simulink model "Model_Refrigeration_ON"  (R2022a)
settings: Solver=VariableStepAuto  StartTime=0.0  StopTime=properties_8(15,2)  FixedStep=properties_8(14,2)  MaxStep=properties_8(14,2)  RelTol=1e-3  AbsTol=1e-3
InitFcn:
  | tube_D = 0.02; % [m] Refrigerant tube diameter
  | duct_W = 0.4; % [m] Air duct width
  | house_L = 4.5; % [m] House length
  | house_W = 3; % [m] House width
  | house_H = 2; % [m] House height
  | roof_pitch = 0; % [deg] Roof pitch
undefined symbols (not defined in the file or in its folder): alpha_h_ratio_NE, alpha_h_ratio_NW, alpha_h_ratio_SE, alpha_h_ratio_SW, area_furniture, area_roof, area_wall_exterior_NE, area_wall_exterior_NW, area_wall_exterior_SE, area_wall_exterior_SW, area_window, cp_furniture, cp_roof, cp_wall_exterior_NE, cp_wall_exterior_NW, cp_wall_exterior_SE, cp_wall_exterior_SW, cp_window, hc_furniture_interior, hc_roof_exterior, hc_roof_interior, hc_wall_exterior_NE, hc_wall_exterior_NW, hc_wall_exterior_SE, hc_wall_exterior_SW, hc_wall_interior_NE, hc_wall_interior_NW, hc_wall_interior_SE, hc_wall_interior_SW, hc_window_exterior, hc_window_interior, k_roof, k_wall_NE, k_wall_NW, k_wall_SE, k_wall_SW, k_window, l_roof, mass_furniture, pitch_roof, properties_8, properties_9, Q_infiltration_latent, Q_infiltration_sensible, Q_latent_occupant_skin, Q_lights, Q_motor, Q_occupant, rho_roof, rho_wall_NE, rho_wall_NW, rho_wall_SE, rho_wall_SW, rho_window, SC, sigbuilder_block, T_env, T_house_init, T_init_furniture, T_set ... (+12)
libraries: fl_lib x102, nesl_utility x30, SimscapeFluids_lib x9, simulink_extras x3
(part 1 of 4)
CloseFcn:
  | try,close(h1_sscfluids_refrigeration),end
  | clear h1_sscfluids_refrigeration
  | try,close(h2_sscfluids_refrigeration),end
  | clear h2_sscfluids_refrigeration
  | try,close(h3_sscfluids_refrigeration),end
  | clear h3_sscfluids_refrigeration
  | Results
  | clear tout simlog_sscfluids_refrigeration
  | clear T_env RH_env T_house_init RH_house_init T_set
  | clear tube_D duct_W house_L house_W house_H roof_pitch
Description:
  | Refrigeration Cycle (Air Conditioning)
settings Model: Creator=The MathWorks, Inc.  LastModifiedBy=Aqib Habib
settings SolverCC: AutoScaleAbsTol=off  AlgebraicLoopSolver=TrustRegion  MaxZcPerStep=1
settings DataIOCC: ReturnWorkspaceOutputs=off
settings DebuggingCC: UnconnectedInputMsg=warning  UnconnectedOutputMsg=warning  UnconnectedLineMsg=warning  SymbolicDimsDataTypeCodeGenerationDiagnostic=none  SFMachineParentedDataDiag=warning
settings SFSimCC: CustomCodeUndefinedFunction=UseInterfaceOnly
settings RTWCC: DLArmComputeVersion=19.05
settings SimscapeCC: SimscapeLogType=all  SimscapeLogSimulationStatistics=on  SimscapeLogName=simlog_sscfluids_refrigeration  SimscapeLogDataHistory=10000

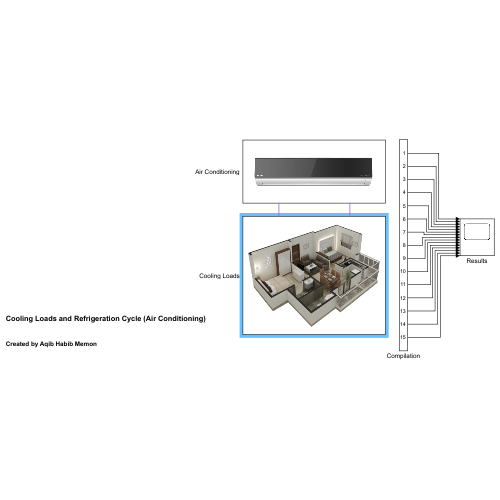
[thumbnail: Simulink's stored preview of the top-level diagram]
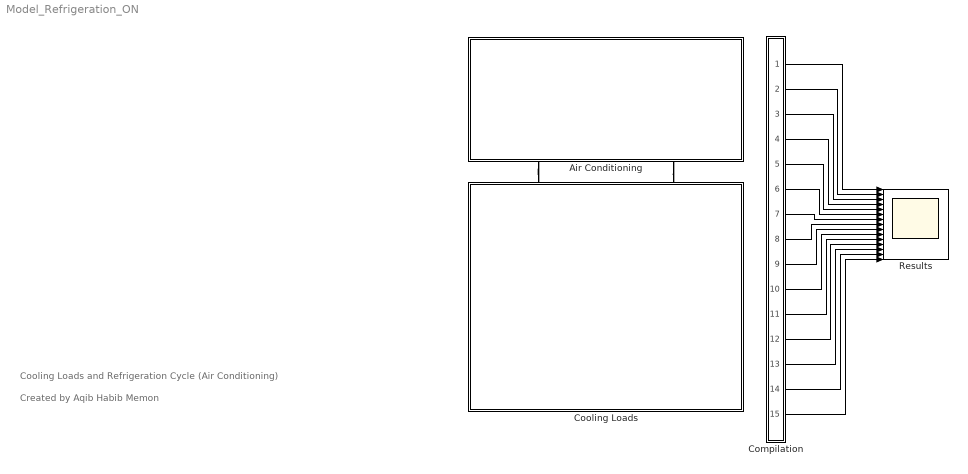
== system Model_Refrigeration_ON ==
  note: Cooling Loads and Refrigeration Cycle (Air Conditioning)
  note: Created by Aqib Habib Memon
  Air Conditioning : Subsystem
      mask Display: image('econo.png'); % Use "Edit Image" on toolstrip to change.
  Compilation : Subsystem
  Cooling Loads : Subsystem
      mask Display: image('Picture1.png'); % Use "Edit Image" on toolstrip to change.
  Results : Scope  NumInputPorts=15
  wires:
  Compilation/10(Out5) -> Results/10
  Compilation/9(Out4) -> Results/9
  Compilation/1(Out1) -> Results/1
  Compilation/2(Out13) -> Results/2
  Compilation/8(Out3) -> Results/8
  Compilation/7(Out7) -> Results/7
  Compilation/12(Out9) -> Results/12
  Compilation/5(Out2) -> Results/5
  Compilation/11(Out8) -> Results/11
  Compilation/6(Out6) -> Results/6
  Compilation/13(Out10) -> Results/13
  Compilation/3(Out12) -> Results/3
  Compilation/4(Out11) -> Results/4
  Compilation/14(Out14) -> Results/14
  Compilation/15(Out15) -> Results/15
  connections:
  Air Conditioning/RConn2 -- Cooling Loads/LConn2
  Air Conditioning/RConn1 -- Cooling Loads/LConn1

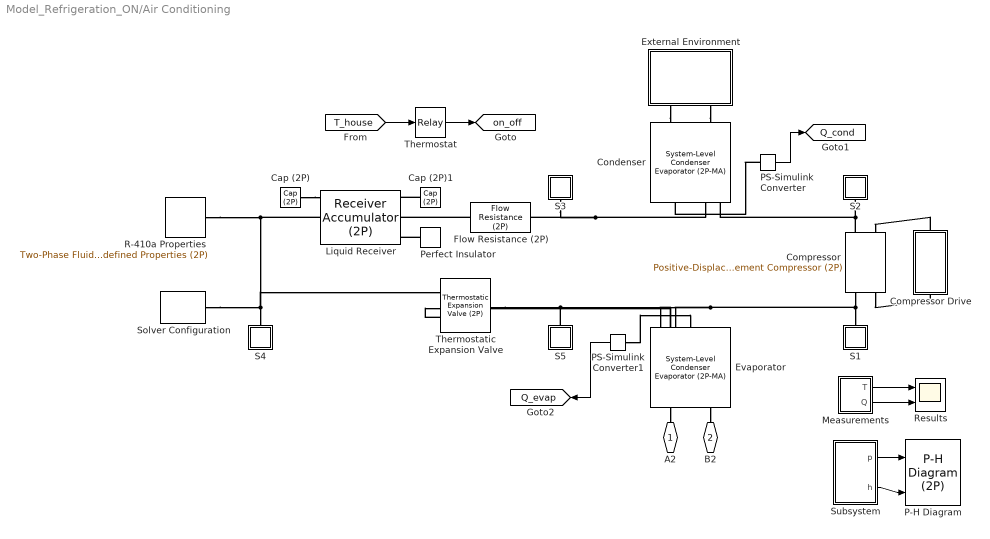
== system Model_Refrigeration_ON/Air Conditioning ==
  Cap (2P) : fl_lib/Two-Phase Fluid/Elements/Cap (2P)  p_specify=off  p_priority=None  p=0.101325 MPa  p_nominal_specify=off  p_nominal_unit=MPa  p_nominal_value=1  u_specify=off  u_priority=None  u=1500 kJ/kg  u_nominal_specify=off  u_nominal_unit=kJ/kg  u_nominal_value=1
      settings: SourceProductBaseCode=PW,SS,VE  InternalSimscapePortConfiguration="{\"Bottom\":[],\"Left\":[{\"id\":\"A\",\"label\":\"\",\"type\":\"foundation.two_phase_fluid.two_phase_fluid\"}],\"Right\":[],\"Top\":[]}"
  Cap (2P)1 : fl_lib/Two-Phase Fluid/Elements/Cap (2P)  p_specify=off  p_priority=None  p=0.101325 MPa  p_nominal_specify=off  p_nominal_unit=MPa  p_nominal_value=1  u_specify=off  u_priority=None  u=1500 kJ/kg  u_nominal_specify=off  u_nominal_unit=kJ/kg  u_nominal_value=1
      settings: SourceProductBaseCode=PW,SS,VE  InternalSimscapePortConfiguration="{\"Bottom\":[],\"Left\":[{\"id\":\"A\",\"label\":\"\",\"type\":\"foundation.two_phase_fluid.two_phase_fluid\"}],\"Right\":[],\"Top\":[]}"
  Compressor : SimscapeFluids_lib/Two-Phase Fluid/Fluid Machines/Positive-Displacement Compressor (2P)  dispSpec=fluids.two_phase_fluid.fluid_machines.enum.DisplacementSpecification.FlowSpeed  v_disp=130 cm^3/rev  mdot_nom=properties_9(1,12) kg/s  omega_nom=properties_9(2,12) rpm  nominalSpec=fluids.two_phase_fluid.fluid_machines.enum.NominalConditionsSpecification.NominalTemps  pr_nom=5  p_in_nom=0.101325 MPa  T_in_nom=373.15 K  T_evap_nom=properties_9(3,12) degC  T_cond_nom=properties_9(4,12) degC  delta_T_nom=properties_9(6,12) deltaK  efficiencySpec=fluids.two_phase_fluid.fluid_machines.enum.VolumetricEfficiencyParameterization.Analytical  eta_nom=properties_9(9,12)  omega_TLU=[800, 1500, 2800, 3300, 4000] rpm  pr_TLU=[2, 4, 6, 8]  eta_TLU=[.95, .9, .85, .8, .75; .925, .875, .825, .775, .725; .875, .825, .775, .725, .675; .75, .7, .65, .6, .55]  n=properties_9(11,12)  mechanical_efficiency=properties_9(10,12)  area_A=pi*properties_9(7,12)/4 m^2  area_B=pi*properties_9(8,12)/4 m^2  VaporCheck=simscape.enum.assert.action.none
      settings: SourceProductBaseCode=SH  InternalSimscapePortConfiguration="{\"Bottom\":[],\"Left\":[{\"id\":\"A\",\"label\":\"A\",\"type\":\"foundation.two_phase_fluid.two_phase_fluid\"},{\"id\":\"C\",\"label\":\"C\",\"type\":\"foundation.mechanical.rotational.rotational\"}],\"Right\":[{\"id\":\"B\",\"label\":\"B\",\"type\":\"foundation.two_phase_fluid.two_phase_fluid\"},{\"id\":\"R\",\"label\":\"R\",\"type\":\"foundation.mechanical.rotational.rotational\"}],\"Top\":[]}"
  Compressor Drive : Subsystem
      settings: PortSchema="{\"entries\":[{\"content\":{\"sides\":[{\"content\":{\"connectorIds\":[]},\"type\":\"ConnectorPlacement.EquallySpacedRectSide\",\"uuid\":\"e1f7673a-ae09-4e38-a748-d03f3a89f634\"},{\"content\":{\"connectorIds\":[],\"side\":\"RIGHT\"},\"type\":\"ConnectorPlacement.EquallySpacedRectSide\",\"uuid\":\"e2c59df4-5a81-4f6b-ab06-631ef800c0b1\"},{\"content\":{\"connectorIds\":[\"LConn1\"],\"side\":\"TOP\"},\"type\":\"ConnectorPlacement.EquallySpacedRectSide\",\"uuid\":\"19dd88a8-04e0-4296-a227-9de66059cdf8\"},{\"content\":{\"connectorIds\":[\"RConn1\"],\"side\":\"BOTTOM\"},\"type\":\"ConnectorPlacement.EquallySpacedRectSide\",\"uuid\":\"d46824c3-70de-4a16-8a6e-f7ccc848533a\"}]},\"type\":\"ConnectorPlacement.EquallySpacedConnector\",\"uuid\":\"cfca4f7e-9c0e-462b-910e-b09b0fceba6e\"}],\"packageUris\":[\"http://schema.mathworks.com/mf0/Connector/R2020b\"],\"version\":\"1.0\"}"
  Condenser : SimscapeFluids_lib/Fluid Network Interfaces/Heat Exchangers/System-Level Condenser Evaporator (2P-MA)  flow_arrangement=fluids.interfaces.heat_exchangers.enum.SystemLevelFlowArrangement2PMA.Cross  wall_thermal_mass=simscape.enum.onoff.off  mass_wall=1 kg  cp_wall=490 J/(K*kg)  area_A1=pi*properties_9(1,4)^2/4 m^2  area_B1=pi*properties_9(2,4)/4 m^2  area_A2=pi*properties_9(3,4)/4 m^2  area_B2=pi*properties_9(4,4)/4 m^2  operating_condition_2P=fluids.interfaces.heat_exchangers.enum.SystemLevelOperatingCondition2PMA.Condenser  mdot_nominal_2P=properties_9(11,4) kg/s  delta_p_nominal_2P=0.01 MPa  pressure_spec_cond_2P=fluids.interfaces.heat_exchangers.enum.SystemLevelPressureSpecCondenser2P.CondensingTemperature  pressure_spec_evap_2P=fluids.interfaces.heat_exchangers.enum.SystemLevelPressureSpecEvaporator2P.InletPressure  p_in_nominal_2P=1 MPa  T_cond_nominal_2P=properties_9(4,12) degC  T_evap_nominal_2P=243.15 K  inlet_spec_2P=fluids.interfaces.heat_exchangers.enum.SystemLevelInletSpec2P.Temperature  T_in_nominal_2P=properties_9(10,4) degC  h_in_nominal_2P=440 kJ/kg  x_in_nominal_2P=1  capacity_spec_2P=fluids.interfaces.heat_exchangers.enum.SystemLevelCapacitySpec.OutletCondition  Q_nominal=0.1 kW  outlet_spec_cond_2P=fluids.interfaces.heat_exchangers.enum.SystemLevelOutletSpecCondenser2P.Subcooling  outlet_spec_evap_2P=fluids.interfaces.heat_exchangers.enum.SystemLevelOutletSpecEvaporator2P.Enthalpy  delta_T_sub_nominal_2P=properties_9(5,12) deltaK  delta_T_sup_nominal_2P=5 deltaK  h_out_nominal_2P=250 kJ/kg  x_out_nominal_2P=0  volume_2P=0.005 m^3  init_spec_2P=fluids.interfaces.heat_exchangers.enum.SystemLevelInitialConditionSpec.Operating  energy_spec_2P=foundation.enum.energy_spec.enthalpy  p_init_2P=0.101325 MPa  T_init_2P=293.15 K  x_init_2P=0.5  alpha_init_2P=0.5  h_init_2P=1500 kJ/kg  u_init_2P=1500 kJ/kg  mdot_nominal_MA=properties_9(5,8) kg/s  delta_p_nominal_MA=200 Pa  p_in_nominal_MA=properties_9(4,8) MPa  T_in_nominal_MA=properties_9(1,8) degC  inlet_moisture_spec_MA=foundation.enum.moisture_spec.relative_humidity  RH_in_nominal_MA=properties_9(2,8)  x_w_in_nominal_MA=0.01  y_w_in_nominal_MA=0.01  HR_in_nominal_MA=0.01  inlet_trace_gas_spec_MA=foundation.enum.trace_gas_spec.mole_fraction  x_g_in_nominal_MA=0.001  y_g_in_nominal_MA=0  volume_MA=properties_9(3,8) m^3  init_spec_MA=fluids.interfaces.heat_exchangers.enum.SystemLevelInitialConditionSpec.Operating  p_init_MA=0.101325 MPa  T_init_MA=293.15 K  moisture_spec_MA=foundation.enum.moisture_spec.relative_humidity  RH_init_MA=0.5  x_w_init_MA=0.01  y_w_init_MA=0.01  HR_init_MA=0.01  trace_gas_spec_MA=foundation.enum.trace_gas_spec.mass_fraction  x_g_init_MA=0.001  y_g_init_MA=0.001  RH_ws_MA=1  a_liq_2P=0.023  a_mix_2P=0.005  a_vap_2P=0.023  b_2P=0.8  c_2P=0.33  a_MA=0.023  b_MA=0.8  c_MA=0.33
      settings: SourceProductBaseCode=SH  InternalSimscapePortConfiguration="{\"Bottom\":[],\"Left\":[{\"id\":\"A1\",\"label\":\"A1\",\"type\":\"foundation.two_phase_fluid.two_phase_fluid\"},{\"id\":\"B1\",\"label\":\"B1\",\"type\":\"foundation.two_phase_fluid.two_phase_fluid\"}],\"Right\":[{\"id\":\"A2\",\"label\":\"A2\",\"type\":\"foundation.moist_air.moist_air\"},{\"id\":\"B2\",\"label\":\"B2\",\"type\":\"foundation.moist_air.moist_air\"}],\"Top\":[{\"id\":\"Q1\",\"label\":\"Q1\",\"type\":\"output\"},{\"id\":\"Q2\",\"label\":\"Q2\",\"type\":\"output\"},{\"id\":\"W\",\"label\":\"W\",\"type\":\"output\"}]}"
  Evaporator : SimscapeFluids_lib/Fluid Network Interfaces/Heat Exchangers/System-Level Condenser Evaporator (2P-MA)  flow_arrangement=fluids.interfaces.heat_exchangers.enum.SystemLevelFlowArrangement2PMA.Cross  wall_thermal_mass=simscape.enum.onoff.off  mass_wall=1 kg  cp_wall=490 J/(K*kg)  area_A1=pi*properties_9(1,2)/4 m^2  area_B1=pi*properties_9(2,2)/4 m^2  area_A2=pi*properties_9(3,2)/4 m^2  area_B2=pi*properties_9(4,2)/4 m^2  operating_condition_2P=fluids.interfaces.heat_exchangers.enum.SystemLevelOperatingCondition2PMA.Evaporator  mdot_nominal_2P=properties_9(11,2) kg/s  delta_p_nominal_2P=0.01 MPa  pressure_spec_cond_2P=fluids.interfaces.heat_exchangers.enum.SystemLevelPressureSpecCondenser2P.InletPressure  pressure_spec_evap_2P=fluids.interfaces.heat_exchangers.enum.SystemLevelPressureSpecEvaporator2P.EvaporatingTemperature  p_in_nominal_2P=1 MPa  T_cond_nominal_2P=313.15 K  T_evap_nominal_2P=properties_9(3,12) degC  inlet_spec_2P=fluids.interfaces.heat_exchangers.enum.SystemLevelInletSpec2P.Enthalpy  T_in_nominal_2P=333.15 K  h_in_nominal_2P=properties_9(8,2) kJ/kg  x_in_nominal_2P=1  capacity_spec_2P=fluids.interfaces.heat_exchangers.enum.SystemLevelCapacitySpec.OutletCondition  Q_nominal=0.1 kW  outlet_spec_cond_2P=fluids.interfaces.heat_exchangers.enum.SystemLevelOutletSpecCondenser2P.Enthalpy  outlet_spec_evap_2P=fluids.interfaces.heat_exchangers.enum.SystemLevelOutletSpecEvaporator2P.Enthalpy  delta_T_sub_nominal_2P=5 deltaK  delta_T_sup_nominal_2P=5 deltaK  h_out_nominal_2P=properties_9(5,2) kJ/kg  x_out_nominal_2P=0  volume_2P=0.005 m^3  init_spec_2P=fluids.interfaces.heat_exchangers.enum.SystemLevelInitialConditionSpec.Operating  energy_spec_2P=foundation.enum.energy_spec.enthalpy  p_init_2P=0.101325 MPa  T_init_2P=293.15 K  x_init_2P=0.5  alpha_init_2P=0.5  h_init_2P=1500 kJ/kg  u_init_2P=1500 kJ/kg  mdot_nominal_MA=properties_9(5,6) kg/s  delta_p_nominal_MA=150 Pa  p_in_nominal_MA=properties_9(4,6) MPa  T_in_nominal_MA=properties_9(1,6) degC  inlet_moisture_spec_MA=foundation.enum.moisture_spec.relative_humidity  RH_in_nominal_MA=properties_9(2,6)  x_w_in_nominal_MA=0.01  y_w_in_nominal_MA=0.01  HR_in_nominal_MA=0.01  inlet_trace_gas_spec_MA=foundation.enum.trace_gas_spec.mole_fraction  x_g_in_nominal_MA=0.001  y_g_in_nominal_MA=0  volume_MA=properties_9(3,6) m^3  init_spec_MA=fluids.interfaces.heat_exchangers.enum.SystemLevelInitialConditionSpec.Operating  p_init_MA=0.101325 MPa  T_init_MA=293.15 K  moisture_spec_MA=foundation.enum.moisture_spec.relative_humidity  RH_init_MA=0.5  x_w_init_MA=0.01  y_w_init_MA=0.01  HR_init_MA=0.01  trace_gas_spec_MA=foundation.enum.trace_gas_spec.mass_fraction  x_g_init_MA=0.001  y_g_init_MA=0.001  RH_ws_MA=1  a_liq_2P=0.023  a_mix_2P=0.005  a_vap_2P=0.023  b_2P=0.8  c_2P=0.33  a_MA=0.023  b_MA=0.8  c_MA=0.33
      settings: SourceProductBaseCode=SH  InternalSimscapePortConfiguration="{\"Bottom\":[],\"Left\":[{\"id\":\"A1\",\"label\":\"A1\",\"type\":\"foundation.two_phase_fluid.two_phase_fluid\"},{\"id\":\"B1\",\"label\":\"B1\",\"type\":\"foundation.two_phase_fluid.two_phase_fluid\"}],\"Right\":[{\"id\":\"A2\",\"label\":\"A2\",\"type\":\"foundation.moist_air.moist_air\"},{\"id\":\"B2\",\"label\":\"B2\",\"type\":\"foundation.moist_air.moist_air\"}],\"Top\":[{\"id\":\"Q1\",\"label\":\"Q1\",\"type\":\"output\"},{\"id\":\"Q2\",\"label\":\"Q2\",\"type\":\"output\"},{\"id\":\"W\",\"label\":\"W\",\"type\":\"output\"}]}"
  External Environment : Subsystem  Tag=PublishSubsystem
      settings: PortSchema="{\"entries\":[{\"content\":{\"sides\":[{\"content\":{\"connectorIds\":[]},\"type\":\"ConnectorPlacement.EquallySpacedRectSide\",\"uuid\":\"e1f7673a-ae09-4e38-a748-d03f3a89f634\"},{\"content\":{\"connectorIds\":[],\"side\":\"RIGHT\"},\"type\":\"ConnectorPlacement.EquallySpacedRectSide\",\"uuid\":\"e2c59df4-5a81-4f6b-ab06-631ef800c0b1\"},{\"content\":{\"connectorIds\":[],\"side\":\"TOP\"},\"type\":\"ConnectorPlacement.EquallySpacedRectSide\",\"uuid\":\"19dd88a8-04e0-4296-a227-9de66059cdf8\"},{\"content\":{\"connectorIds\":[\"RConn1\",\"RConn2\"],\"side\":\"BOTTOM\"},\"type\":\"ConnectorPlacement.EquallySpacedRectSide\",\"uuid\":\"7fa7b35b-dcaf-4306-877d-c86d73f259c8\"}]},\"type\":\"ConnectorPlacement.EquallySpacedConnector\",\"uuid\":\"cfca4f7e-9c0e-462b-910e-b09b0fceba6e\"}],\"packageUris\":[\"http://schema.mathworks.com/mf0/Connector/R2020b\"],\"version\":\"1.0\"}"
      mask Display: image('en-ca-house-summer_0.jpg'); % Use "Edit Image" on toolstrip to change.
  Flow Resistance (2P) : fl_lib/Two-Phase Fluid/Elements/Flow Resistance (2P)  delta_p_nominal=0.05 MPa  mdot_nominal=0.1 kg/s  v_nominal=0 m^3/kg  area=pi*tube_D^2/4 m^2  laminar_fraction=1e-3
      settings: SourceProductBaseCode=PW,SS,VE  InternalSimscapePortConfiguration="{\"Bottom\":[],\"Left\":[{\"id\":\"A\",\"label\":\"A\",\"type\":\"foundation.two_phase_fluid.two_phase_fluid\"}],\"Right\":[{\"id\":\"B\",\"label\":\"B\",\"type\":\"foundation.two_phase_fluid.two_phase_fluid\"}],\"Top\":[]}"
  Liquid Receiver : SimscapeFluids_lib/Two-Phase Fluid/Tanks & Accumulators/Receiver Accumulator (2P)  volume=properties_9(1,10) m^3  tank_area=properties_9(2,10) m^2  area_AV=pi*tube_D^2/4 m^2  area_BV=pi*tube_D^2/4 m^2  area_AL=pi*properties_9(3,10)^2/4 m^2  area_BL=pi*properties_9(4,10)^2/4 m^2  V_frac_error=simscape.enum.assert.action.none  V_frac_min=0.05  V_frac_max=0.95  V_frac_smooth=0.05  p_crit_error=simscape.enum.assert.action.error  hc_vap=20 W/(K*m^2)  hc_liq=100 W/(K*m^2)  receiver_accumulator_energy_spec=fluids.two_phase_fluid.enum.receiver_accumulator_energy_spec.volume_fraction  p_init=properties_9(5,10) MPa  T_init=293.15 K  M_frac_init=0.5  V_frac_init=properties_9(6,10)  h_init=1500 kJ/kg  u_init=1500 kJ/kg  tau_vap_cond=1 s
      settings: SourceProductBaseCode=SH  InternalSimscapePortConfiguration="{\"Bottom\":[],\"Left\":[{\"id\":\"AV\",\"label\":\"AV\",\"type\":\"foundation.two_phase_fluid.two_phase_fluid\"},{\"id\":\"AL\",\"label\":\"AL\",\"type\":\"foundation.two_phase_fluid.two_phase_fluid\"},{\"id\":\"H\",\"label\":\"H\",\"type\":\"foundation.thermal.thermal\"}],\"Right\":[{\"id\":\"BV\",\"label\":\"BV\",\"type\":\"foundation.two_phase_fluid.two_phase_fluid\"},{\"id\":\"BL\",\"label\":\"BL\",\"type\":\"foundation.two_phase_fluid.two_phase_fluid\"},{\"id\":\"L\",\"label\":\"L\",\"type\":\"output\"}],\"Top\":[]}"
  Measurements : Subsystem
  P-H Diagram : SimscapeFluids_lib/Two-Phase Fluid/Utilities/P-H Diagram (2P)
      settings: SourceProductBaseCode=SH
  PS-Simulink Converter : nesl_utility/PS-Simulink Converter  PhysicalDomain=network_engine_domain  SubClassName=ps_output  LeftPortType=input  RightPortType=output  PseudoPeriodic=off  Frequencies=[]  VectorFormat=inherit  Unit=W  AffineConversion=off
      settings: SourceProductBaseCode=SS,PW,VE
  PS-Simulink Converter1 : nesl_utility/PS-Simulink Converter  PhysicalDomain=network_engine_domain  SubClassName=ps_output  LeftPortType=input  RightPortType=output  PseudoPeriodic=off  Frequencies=[]  VectorFormat=inherit  Unit=W  AffineConversion=off
      settings: SourceProductBaseCode=SS,PW,VE
  Perfect Insulator : fl_lib/Thermal/Thermal Elements/Perfect Insulator  T_specify=off  T_priority=None  T=293.15 K  T_nominal_specify=off  T_nominal_unit=K  T_nominal_value=1
      settings: SourceProductBaseCode=PW,SS,VE
  R-410a Properties : SimscapeFluids_lib/Two-Phase Fluid/Utilities/Two-Phase Fluid Predefined Properties (2P)  fluid=fluids.two_phase_fluid.utilities.enum.Fluid.R410a  p_atm=0.101325 MPa  q_rev=0.01 Pa
      settings: SourceProductBaseCode=SH
  Results : Scope  NumInputPorts=2
  S1 : Subsystem
      mask Display: disp(get_param(gcb, 'Name'))
  S2 : Subsystem
      mask Display: disp(get_param(gcb, 'Name'))
  S3 : Subsystem
      mask Display: disp(get_param(gcb, 'Name'))
  S4 : Subsystem
      mask Display: disp(get_param(gcb, 'Name'))
  S5 : Subsystem
      mask Display: disp(get_param(gcb, 'Name'))
  Solver Configuration : nesl_utility/Solver Configuration  PhysicalDomain=network_engine_domain  SubClassName=solver  LeftPortType=input  RightPortType=generic  Tones=[]  Harmonics=[]  SimulateNoise=off  Profile=off  UseLocalSampling=off  EnableSwitchedLinearOptims=on  FrequencyDomain=off  UseCCode=off  RelTol=0.001  AbsTol=0.001  MinStep=1e-09  ToWorkspace=off  RevertToSquareIcSolve=off  NumHomotopyIterations=100  PhasorMode=off  PhasorModeNumHarmonics=1  IndexReductionMethod=DerivativeReplacement  DoDC=off  ResidualTolerance=1e-09  UseLocalSolver=off  LocalSolverChoice=NE_BACKWARD_EULER_ADVANCER  LocalSolverSampleTime=0.001  DoFixedCost=off  MaxNonlinIter=3  MaxModeIter=2  ComputeImpulses=off  ImpulseIterations=2  LinearAlgebra=auto  LinearAlgebraNumThread=0  EquationFormulation=NE_TIME_EF  DelaysMemoryBudget=1024  AutomaticFiltering=on  FilteringTimeConstant=0.001  PartitionStorageMethod=AS_NEEDED  PartitionMemoryBudget=1024  PartitionMethod=ROBUST
      settings: SourceProductBaseCode=SS,PW,VE
  Subsystem : Subsystem
  Thermostat : Relay  OnSwitchValue=T_set + 1  OffSwitchValue=T_set - 1  ZeroCross=off
  Thermostatic Expansion Valve : SimscapeFluids_lib/Two-Phase Fluid/Valves & Orifices/Flow Control Valves/Thermostatic Expansion Valve (2P)  Q_nominal=properties_9(1,14) kW  Q_max=properties_9(2,14) kW  T_evap=properties_9(3,12) degC  delta_T_static=2 deltaK  delta_T_nominal=5 deltaK  T_cond=properties_9(4,12) degC  delta_T_sub=5 deltaK  pressure_equalization=fluids.two_phase_fluid.valves_orifices.flow_control_valves.enum.ThermostaticExpansionValveEqualization.Internal  mop=fluids.two_phase_fluid.valves_orifices.flow_control_valves.enum.ThermostaticExpansionValveMOP.Off  p_mop=0.5 MPa  T_mop=288.15 K  bulb_dynamics=simscape.enum.onoff.off  tau_bulb=20 s  area=pi*tube_D^2/4 m^2  mdot_leak_fraction=1e-6  smoothing_factor=0.01  B_lam=0.999  tau_x=0.1 s
      settings: SourceProductBaseCode=SH  InternalSimscapePortConfiguration="{\"Bottom\":[],\"Left\":[{\"id\":\"A\",\"label\":\"A\",\"type\":\"foundation.two_phase_fluid.two_phase_fluid\"}],\"Right\":[{\"id\":\"B\",\"label\":\"B\",\"type\":\"foundation.two_phase_fluid.two_phase_fluid\"}],\"Top\":[{\"id\":\"S\",\"label\":\"S\",\"type\":\"foundation.two_phase_fluid.two_phase_fluid\"}]}"
  A2 : PMIOPort  Side=Right
  B2 : PMIOPort  Port=2  Side=Right
  tag scope: Q_cond=global, Q_evap=global, on_off=global
  wires:
  [T_house] -> Thermostat/1
  PS-Simulink Converter1/1 -> [Q_evap]
  Thermostat/1 -> [on_off]
  PS-Simulink Converter/1 -> [Q_cond]
  Measurements/2(Q) -> Results/2
  Measurements/1(T) -> Results/1
  Subsystem/1(p) -> P-H Diagram/1
  Subsystem/2(h) -> P-H Diagram/2
  connections:
  Thermostatic Expansion Valve/RConn1 -- Evaporator/LConn1 -- S5/LConn1
  Liquid Receiver/RConn2 -- R-410a Properties/RConn1 -- Thermostatic Expansion Valve/LConn1 -- S4/LConn1 -- Solver Configuration/RConn1
  External Environment/RConn1 -- Condenser/RConn2
  Flow Resistance (2P)/RConn1 -- Liquid Receiver/LConn2
  Cap (2P)/LConn1 -- Liquid Receiver/RConn1
  Evaporator/RConn1 -- A2/RConn1
  Cap (2P)1/LConn1 -- Liquid Receiver/LConn1
  Compressor/RConn1 -- Condenser/LConn1 -- S2/LConn1
  Condenser/LConn2 -- Flow Resistance (2P)/LConn1 -- S3/LConn1
  Perfect Insulator/LConn1 -- Liquid Receiver/LConn3
  Compressor/LConn1 -- Evaporator/LConn2 -- Thermostatic Expansion Valve/LConn2 -- S1/LConn1
  Evaporator/RConn2 -- B2/RConn1
  Compressor Drive/LConn1 -- Compressor/RConn2
  Compressor/LConn2 -- Compressor Drive/RConn1
  External Environment/RConn2 -- Condenser/RConn1
  PS-Simulink Converter/LConn1 -- Condenser/LConn4
  PS-Simulink Converter1/LConn1 -- Evaporator/LConn3

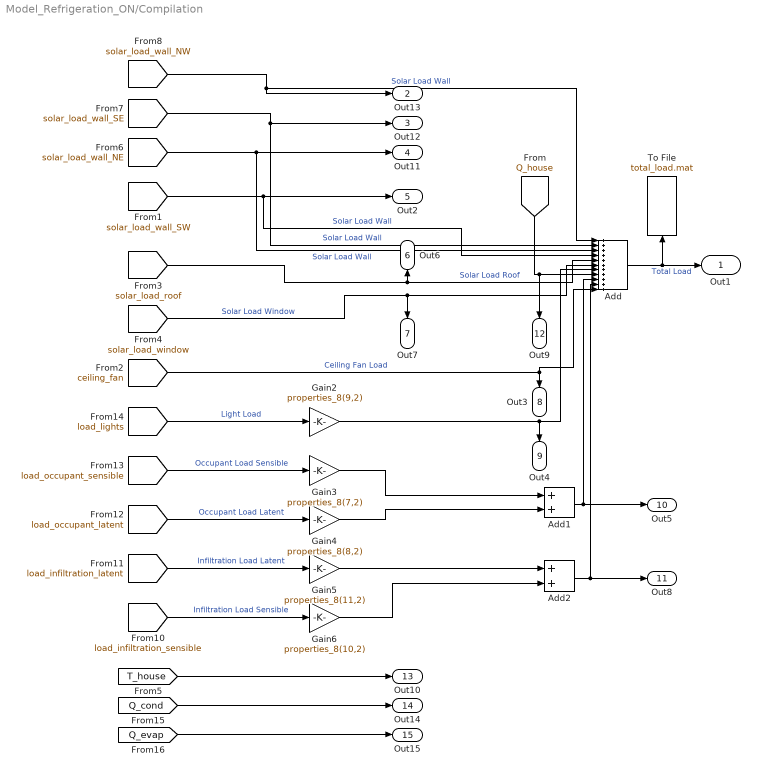
== system Model_Refrigeration_ON/Compilation ==
  Add : Sum  Inputs=+++++++++++
  Add1 : Sum
  Add2 : Sum
  Gain2 : Gain  Gain=properties_8(9,2)
  Gain3 : Gain  Gain=properties_8(7,2)
  Gain4 : Gain  Gain=properties_8(8,2)
  Gain5 : Gain  Gain=properties_8(11,2)
  Gain6 : Gain  Gain=properties_8(10,2)
  To File : ToFile  Filename=total_load.mat  MatrixName=total_load
  Out1 : Outport
  Out13 : Outport  Port=2
  Out12 : Outport  Port=3
  Out11 : Outport  Port=4
  Out2 : Outport  Port=5
  Out6 : Outport  Port=6
  Out7 : Outport  Port=7
  Out3 : Outport  Port=8
  Out4 : Outport  Port=9
  Out5 : Outport  Port=10
  Out8 : Outport  Port=11
  Out9 : Outport  Port=12
  Out10 : Outport  Port=13
  Out14 : Outport  Port=14
  Out15 : Outport  Port=15
  wires:
  [load_lights] -> Gain2/1  "Light Load"
  [ceiling_fan] -> Add/11, Out3/1  "Ceiling Fan Load"
  [load_occupant_sensible] -> Gain3/1  "Occupant Load Sensible"
  [load_occupant_latent] -> Gain4/1  "Occupant Load Latent"
  [load_infiltration_sensible] -> Gain6/1  "Infiltration Load Sensible"
  [Q_house] -> Add/8, Out9/1
  [solar_load_wall_SW] -> Add/4, Out2/1  "Solar Load Wall"
  [solar_load_roof] -> Add/5, Out6/1  "Solar Load Roof"
  [solar_load_window] -> Add/6, Out7/1  "Solar Load Window"
  [T_house] -> Out10/1
  [solar_load_wall_NE] -> Add/3, Out11/1  "Solar Load Wall"
  [solar_load_wall_SE] -> Add/2, Out12/1  "Solar Load Wall"
  [solar_load_wall_NW] -> Add/1, Out13/1  "Solar Load Wall"
  [load_infiltration_latent] -> Gain5/1  "Infiltration Load Latent"
  Add1/1 -> Out5/1, Add/9
  Add2/1 -> Add/10, Out8/1
  Gain2/1 -> Add/7, Out4/1
  Gain3/1 -> Add1/1
  Gain4/1 -> Add1/2
  Gain5/1 -> Add2/1
  Gain6/1 -> Add2/2
  [Q_evap] -> Out15/1
  [Q_cond] -> Out14/1
  Add/1 -> To File/1, Out1/1  "Total Load"

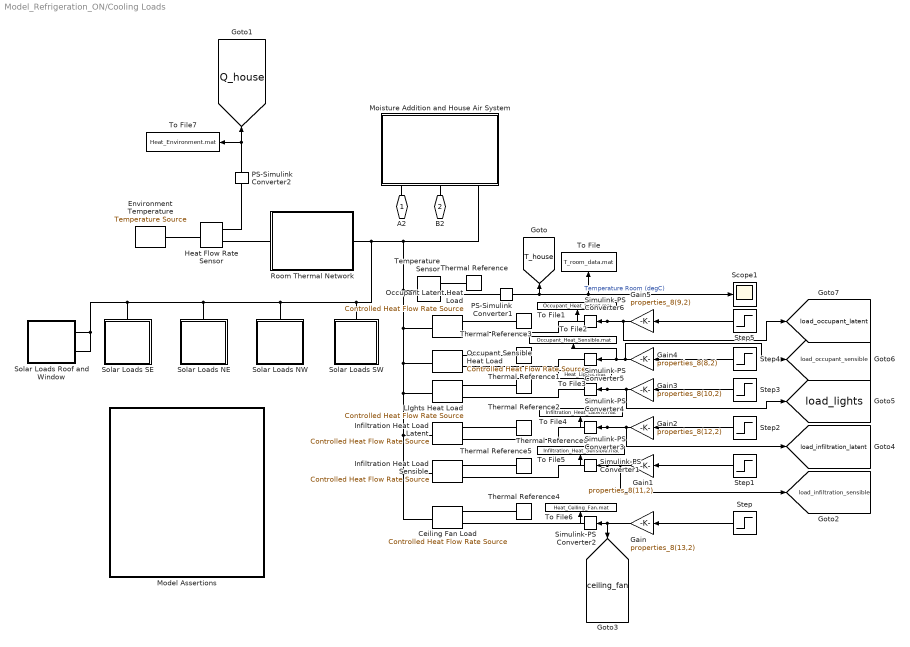
== system Model_Refrigeration_ON/Cooling Loads ==
  Ceiling Fan Load : fl_lib/Thermal/Thermal Sources/Controlled Heat Flow Rate Source
      settings: SourceProductBaseCode=PW,SS,VE
  Environment Temperature : fl_lib/Thermal/Thermal Sources/Temperature Source  temperature=T_env degC
      settings: SourceProductBaseCode=PW,SS,VE
  Gain : Gain  Gain=properties_8(13,2)
  Gain1 : Gain  Gain=properties_8(11,2)
  Gain2 : Gain  Gain=properties_8(12,2)
  Gain3 : Gain  Gain=properties_8(10,2)
  Gain4 : Gain  Gain=properties_8(8,2)
  Gain5 : Gain  Gain=properties_8(9,2)
  Heat Flow Rate Sensor : fl_lib/Thermal/Thermal Sensors/Heat Flow Rate Sensor
      settings: SourceProductBaseCode=PW,SS,VE
  Infiltration Heat Load Latent : fl_lib/Thermal/Thermal Sources/Controlled Heat Flow Rate Source
      settings: SourceProductBaseCode=PW,SS,VE
  Infiltration Heat Load Sensible : fl_lib/Thermal/Thermal Sources/Controlled Heat Flow Rate Source
      settings: SourceProductBaseCode=PW,SS,VE
  LIghts Heat Load : fl_lib/Thermal/Thermal Sources/Controlled Heat Flow Rate Source
      settings: SourceProductBaseCode=PW,SS,VE
  Model Assertions : Subsystem
      mask Display: image('istockphoto-1156490264-612x612.jpg'); % Use "Edit Image" on toolstrip to change.
  Moisture Addition and House Air System : Subsystem
      mask Display: image('pexels-photo-1028600.jpeg'); % Use "Edit Image" on toolstrip to change.
  Occupant Latent Heat Load : fl_lib/Thermal/Thermal Sources/Controlled Heat Flow Rate Source
      settings: SourceProductBaseCode=PW,SS,VE
  Occupant Sensible Heat Load : fl_lib/Thermal/Thermal Sources/Controlled Heat Flow Rate Source
      settings: SourceProductBaseCode=PW,SS,VE
  PS-Simulink Converter1 : nesl_utility/PS-Simulink Converter  PhysicalDomain=network_engine_domain  SubClassName=ps_output  LeftPortType=input  RightPortType=output  PseudoPeriodic=off  Frequencies=[]  VectorFormat=inherit  Unit=degC  AffineConversion=on
      settings: SourceProductBaseCode=SS,PW,VE
  PS-Simulink Converter2 : nesl_utility/PS-Simulink Converter  PhysicalDomain=network_engine_domain  SubClassName=ps_output  LeftPortType=input  RightPortType=output  PseudoPeriodic=off  Frequencies=[]  VectorFormat=inherit  Unit=W  AffineConversion=off
      settings: SourceProductBaseCode=SS,PW,VE
  Room Thermal Network : Subsystem  Tag=PublishSubsystem  mask(House Thermal Network){area_roof=l_roof * w_roof / (2*cosd(pitch_roof)), thickness_roof=thicnkess_roof, rho_roof=rho_roof, cp_roof=cp_roof, k_roof=k_roof, hc_roof_interior=hc_roof_interior, hc_roof_exterior=hc_roof_exterior, T_init_roof=T_house_init, area_wall_SE=area_wall_exterior_SE, thickness_wall_SE=thicnkess_wall_exterior_SE, rho_wall_SE=rho_wall_SE, cp_wall_SE=cp_wall_exterior_SE, k_wall_SE=k_wall_SE, hc_wall_interior_SE=hc_wall_interior_SE, hc_wall_exterior_SE=hc_wall_exterior_SE, T_init_wall_SE=T_house_init, area_wall_NE=area_wall_exterior_NE, thickness_wall_copy_NE=thicnkess_wall_exterior_NE, rho_wall_NE=rho_wall_NE, cp_wall_NE=cp_wall_exterior_NE, k_wall_NE=k_wall_NE, hc_wall_interior_NE=hc_wall_interior_NE, hc_wall_exterior_NE=hc_wall_exterior_NE, T_init_wall_NE=T_house_init, area_wall_SW=area_wall_exterior_SW, thickness_wall_SW=thicnkess_wall_exterior_SW, rho_wal_SW=rho_wall_SW, cp_wall_SW=cp_wall_exterior_SW, k_wall_SW=k_wall_SW, hc_wall_SW=hc_wall_interior_SW, hc_wall_exterior_SW=hc_wall_exterior_SW, T_init_wall_SW=T_house_init, area_wall_NW=area_wall_exterior_NW, thickness_wall_NW=thicnkess_wall_exterior_NW, rho_wall_NW=rho_wall_NW, cp_wall_NW=cp_wall_exterior_NW, k_wall_NW=k_wall_NW, hc_wall_interior_NW=hc_wall_interior_NW, hc_wall_exterior_NW=hc_wall_exterior_NW, T_init_wall_NW=T_house_init, area_window=area_window, thickness_window=thicnkess_window, rho_window=rho_window, cp_window=cp_window, k_window=k_window, hc_window_interior=hc_window_interior, hc_window_exterior=hc_window_exterior, T_init_window=T_house_init, area_furniture=area_furniture, M_furniture=mass_furniture, cp_furniture=cp_furniture, hc_furniture_interior=hc_furniture_interior, T_init_furniture=T_init_furniture}
      mask prompts: area_roof "Total area (m^2)"; thickness_roof "Average thickness (m)"; rho_roof "Average density (kg/m^3)"; cp_roof "Average specific heat (J/kg/K)"; k_roof "Average conductivity (W/m/K)"; hc_roof_interior "Interior heat transfer coefficient (W/m^2/K)"; hc_roof_exterior "Exterior heat transfer coefficient (W/m^2/K)"; T_init_roof "Initial temperature (degC)"; area_wall_SE "Total area (m^2)"; thickness_wall_SE "Average thickness (m)"; rho_wall_SE "Average density (kg/m^3)"; cp_wall_SE "Average specific heat (J/kg/K)"; k_wall_SE "Average conductivity (W/m/K)"; hc_wall_interior_SE "Interior heat transfer coefficient (W/m^2/K)"; hc_wall_exterior_SE "Exterior heat transfer coefficient (W/m^2/K)"; T_init_wall_SE "Initial temperature (degC)"; area_wall_NE "Total area (m^2)"; thickness_wall_copy_NE "Average thickness (m)"; rho_wall_NE "Average density (kg/m^3)"; cp_wall_NE "Average specific heat (J/kg/K)"; k_wall_NE "Average conductivity (W/m/K)"; hc_wall_interior_NE "Interior heat transfer coefficient (W/m^2/K)"; hc_wall_exterior_NE "Exterior heat transfer coefficient (W/m^2/K)"; T_init_wall_NE "Initial temperature (degC)"; area_wall_SW "Total area (m^2)"; thickness_wall_SW "Average thickness (m)"; rho_wal_SW "Average density (kg/m^3)"; cp_wall_SW "Average specific heat (J/kg/K)"; k_wall_SW "Average conductivity (W/m/K)"; hc_wall_SW "Interior heat transfer coefficient (W/m^2/K)"; hc_wall_exterior_SW "Exterior heat transfer coefficient (W/m^2/K)"; T_init_wall_SW "Initial temperature (degC)"; area_wall_NW "Total area (m^2)"; thickness_wall_NW "Average thickness (m)"; rho_wall_NW "Average density (kg/m^3)"; cp_wall_NW "Average specific heat (J/kg/K)"; k_wall_NW "Average conductivity (W/m/K)"; hc_wall_interior_NW "Interior heat transfer coefficient (W/m^2/K)"; hc_wall_exterior_NW "Exterior heat transfer coefficient (W/m^2/K)"; T_init_wall_NW "Initial temperature (degC)"; area_window "Total area (m^2)"; thickness_window "Average thickness (m)"; rho_window "Average density (kg/m^3)"; cp_window "Average specific heat (J/kg/K)"; k_window "Average conductivity (W/m/K)"; hc_window_interior "Interior heat transfer coefficient (W/m^2/K)"; hc_window_exterior "Exterior heat transfer coefficient (W/m^2/K)"; T_init_window "Initial temperature (degC)"; area_furniture "Total surface area (m^2)"; M_furniture "Total mass (kg)"; cp_furniture "Average specific heat (J/kg/K)"; hc_furniture_interior "Interior heat transfer coefficient (W/m^2/K)"; T_init_furniture "Initial temperature (degC)"
      mask help: This subsystem models heat transfer between the air in the interior of the house and the external environment.
      mask DialogControl TabRoof Prompt: Roof
      mask DialogControl TabWallSE Prompt: South East Walls
      mask DialogControl TabWallNE Prompt: North East Walls
      mask DialogControl TabWallSW Prompt: South West Walls
      mask DialogControl TabWallNW Prompt: North West Walls
      mask DialogControl TabWindow Prompt: Windows
      mask DialogControl TabFurniture Prompt: Furniture
      mask Display: image('Picture2.png'); % Use "Edit Image" on toolstrip to change.
  Scope1 : Scope
  Simulink-PS Converter{1..6} (6 alike) : nesl_utility/Simulink-PS Converter  PhysicalDomain=network_engine_domain  SubClassName=ps_input  LeftPortType=input  RightPortType=output  PseudoPeriodic=off  Frequencies=[]  NoiseDistribution=none  NoiseParameters=[]  Unit=1  AffineConversion=off  FilteringAndDerivatives=provide  SimscapeFilterOrder=1  InputFilterTimeConstant=0.001  UdotUserProvided=0
      settings: SourceProductBaseCode=SS,PW,VE
  Solar Loads NE : Subsystem
      mask Display: image('sun_048.jpg'); % Use "Edit Image" on toolstrip to change.
  Solar Loads NW : Subsystem
      mask Display: image('sun_048.jpg'); % Use "Edit Image" on toolstrip to change.
  Solar Loads Roof and Window : Subsystem
      mask Display: image('sun_048.jpg'); % Use "Edit Image" on toolstrip to change.
  Solar Loads SE : Subsystem
      mask Display: image('sun_048.jpg'); % Use "Edit Image" on toolstrip to change.
  Solar Loads SW : Subsystem
      mask Display: image('sun_048.jpg'); % Use "Edit Image" on toolstrip to change.
  Step : Step  Time=0  After=Q_motor  SampleTime=0
  Step1 : Step  Time=0  After=Q_infiltration_sensible  SampleTime=0
  Step2 : Step  Time=0  After=Q_infiltration_latent  SampleTime=0
  Step3 : Step  Time=0  After=Q_lights  SampleTime=0
  Step4 : Step  Time=0  After=Q_occupant  SampleTime=0
  Step5 : Step  Time=0  After=Q_latent_occupant_skin  SampleTime=0
  Temperature Sensor : fl_lib/Thermal/Thermal Sensors/Temperature Sensor
      settings: SourceProductBaseCode=PW,SS,VE
  Thermal Reference{,1..6} (7 alike) : fl_lib/Thermal/Thermal Elements/Thermal Reference
      settings: SourceProductBaseCode=PW,SS,VE
  To File : ToFile  Filename=T_room_data.mat  MatrixName=T_room_data
  To File1 : ToFile  Filename=Occupant_Heat_Latent.mat  MatrixName=Occupant_Heat_Latent
  To File2 : ToFile  Filename=Occupant_Heat_Sensible.mat  MatrixName=Occupant_Heat_Sensible
  To File3 : ToFile  Filename=Heat_Lights.mat  MatrixName=Heat_Lights
  To File4 : ToFile  Filename=Infiltration_Heat_Latent.mat  MatrixName=Infiltration_Heat_Latent
  To File5 : ToFile  Filename=Infiltration_Heat_Sensible.mat  MatrixName=Infiltration_Heat_Sensible
  To File6 : ToFile  Filename=Heat_Ceiling_Fan.mat  MatrixName=Heat_Ceiling_Fan
  To File7 : ToFile  Filename=Heat_Environment.mat  MatrixName=Heat_Environment
  A2 : PMIOPort  Side=Left
  B2 : PMIOPort  Port=2  Side=Left
  tag scope: Q_house=global, T_house=global, ceiling_fan=global, load_infiltration_latent=global, load_infiltration_sensible=global, load_lights=global, load_occupant_latent=global, load_occupant_sensible=global
  wires:
  PS-Simulink Converter1/1 -> Scope1/1, To File/1, [T_house]  "Temperature Room (degC)"
  PS-Simulink Converter2/1 -> To File7/1, [Q_house]
  Gain/1 -> To File6/1, [ceiling_fan], Simulink-PS Converter2/1
  Step/1 -> Gain/1
  Step1/1 -> Gain1/1
  Step2/1 -> Gain2/1
  Step3/1 -> Gain3/1
  Step4/1 -> Gain4/1
  Step5/1 -> Gain5/1
  Gain5/1 -> Simulink-PS Converter6/1, To File1/1, [load_occupant_latent]
  Gain3/1 -> [load_lights], To File3/1, Simulink-PS Converter4/1
  Gain2/1 -> [load_infiltration_latent], To File4/1, Simulink-PS Converter3/1
  Gain1/1 -> [load_infiltration_sensible], To File5/1, Simulink-PS Converter1/1
  Gain4/1 -> Simulink-PS Converter5/1, To File2/1, [load_occupant_sensible]
  connections:
  Temperature Sensor/RConn2 -- PS-Simulink Converter1/LConn1
  Temperature Sensor/RConn1 -- Thermal Reference/LConn1
  Moisture Addition and House Air System/LConn3 -- Solar Loads Roof and Window/RConn2 -- Solar Loads Roof and Window/RConn1 -- Solar Loads SE/RConn1 -- Solar Loads NE/RConn1 -- Solar Loads NW/RConn1 -- Solar Loads SW/RConn1 -- Room Thermal Network/RConn1 -- Ceiling Fan Load/LConn1 -- Infiltration Heat Load Sensible/LConn1 -- Infiltration Heat Load Latent/LConn1 -- LIghts Heat Load/LConn1 -- Occupant Sensible Heat Load/LConn1 -- Occupant Latent Heat Load/LConn1 -- Temperature Sensor/LConn1
  Thermal Reference4/LConn1 -- Ceiling Fan Load/RConn2
  Simulink-PS Converter2/RConn1 -- Ceiling Fan Load/RConn1
  Heat Flow Rate Sensor/LConn1 -- Environment Temperature/LConn1
  PS-Simulink Converter2/LConn1 -- Heat Flow Rate Sensor/RConn1
  Occupant Latent Heat Load/RConn2 -- Thermal Reference3/LConn1
  Occupant Sensible Heat Load/RConn2 -- Thermal Reference1/LConn1
  LIghts Heat Load/RConn2 -- Thermal Reference2/LConn1
  Infiltration Heat Load Sensible/RConn2 -- Thermal Reference5/LConn1
  Thermal Reference6/LConn1 -- Infiltration Heat Load Latent/RConn2
  Simulink-PS Converter6/RConn1 -- Occupant Latent Heat Load/RConn1
  Simulink-PS Converter5/RConn1 -- Occupant Sensible Heat Load/RConn1
  Simulink-PS Converter4/RConn1 -- LIghts Heat Load/RConn1
  Simulink-PS Converter3/RConn1 -- Infiltration Heat Load Latent/RConn1
  Simulink-PS Converter1/RConn1 -- Infiltration Heat Load Sensible/RConn1
  Heat Flow Rate Sensor/RConn2 -- Room Thermal Network/LConn1
  A2/RConn1 -- Moisture Addition and House Air System/LConn1
  B2/RConn1 -- Moisture Addition and House Air System/LConn2

== system Model_Refrigeration_ON/Air Conditioning/Compressor Drive ==
  Ideal Angular Velocity Source : fl_lib/Mechanical/Mechanical Sources/Ideal Angular Velocity Source
      settings: SourceProductBaseCode=PW,SS,VE
  Mechanical Rotational Reference : fl_lib/Mechanical/Rotational Elements/Mechanical Rotational Reference
      settings: SourceProductBaseCode=PW,SS,VE
  Shaft Speed : fl_lib/Physical Signals/Functions/PS Gain  gain=1000 rpm
      settings: SourceProductBaseCode=PW,SS,VE
  Simulink-PS Converter : nesl_utility/Simulink-PS Converter  PhysicalDomain=network_engine_domain  SubClassName=ps_input  LeftPortType=input  RightPortType=output  PseudoPeriodic=off  Frequencies=[]  NoiseDistribution=none  NoiseParameters=[]  Unit=1  AffineConversion=off  FilteringAndDerivatives=provide  SimscapeFilterOrder=1  InputFilterTimeConstant=0.001  UdotUserProvided=0
      settings: SourceProductBaseCode=SS,PW,VE
  Transfer Fcn (with initial outputs) : simulink_extras/Additional Linear/Transfer Fcn (with initial outputs)  N=[1]  D="[2  1]"  Y0=1  U0=0
  R : PMIOPort  Side=Left
  C : PMIOPort  Port=2  Side=Right
  wires:
  Transfer Fcn (with initial outputs)/1 -> Simulink-PS Converter/1
  [on_off] -> Transfer Fcn (with initial outputs)/1
  connections:
  Ideal Angular Velocity Source/LConn1 -- R/RConn1
  Ideal Angular Velocity Source/RConn2 -- Mechanical Rotational Reference/LConn1 -- C/RConn1
  Shaft Speed/RConn1 -- Ideal Angular Velocity Source/RConn1
  Simulink-PS Converter/RConn1 -- Shaft Speed/LConn1
